simulink model "closed_loop_system_modal_kp_kv_robustness"  (R2022a)
settings: Solver=ode45  StartTime=0.0  StopTime=10.0  RelTol=1e-3  EnableMultiTasking=on
values from neighbouring files (symbols this model uses):
  Jpl = 0.0124    [lead_compensator.m]    (also in open_loop_complete_system_analysis.m; poles_placement_kp_kv.m; poles_placement_kp_kv_int.m)
  k = 1    [lead_compensator.m]    (also in poles_placement_kp_kv.m = place(openloop_modal_ss.a,openloop_modal_ss.b,lambda); poles_placement_kp_kv_int.m = place(openloop_modal_int_ss.a,openloop_modal_int_ss.b,lambda)
  km = 0.0235    [lead_compensator.m]    (also in open_loop_complete_system_analysis.m; poles_placement_kp_kv.m; poles_placement_kp_kv_int.m)
settings Model: Creator=c.ponzoni  LastModifiedBy=fades
settings SolverCC: AlgebraicLoopSolver=TrustRegion
settings DataIOCC: LimitDataPoints=on  SaveFormat=Array  ReturnWorkspaceOutputs=off
settings OptimizationCC: ExpressionDepthLimit=2147483647  LifeSpan=inf
settings DebuggingCC: UnderspecifiedInitializationDetection=Classic  MergeDetectMultiDrivingBlocksExec=none  UnconnectedInputMsg=warning  UnconnectedOutputMsg=warning  UnconnectedLineMsg=warning  StateNameClashWarn=warning  SFUnexpectedBacktrackingDiag=warning  SFNoUnconditionalDefaultTransitionDiag=warning  SFExecutionAtInitializationDiag=none  SFMachineParentedDataDiag=warning  ArithmeticOperatorsInVariantConditions=warning
settings HardwareCC: ProdBitPerPointer=32  ProdBitPerSizeT=32  ProdBitPerPtrDiffT=32  ProdLargestAtomicFloat=None  ProdIntDivRoundTo=Undefined  ProdEndianess=Unspecified  ProdWordSize=32  ProdHWDeviceType=32-bit Generic
settings ModelReferenceCC: PropagateSignalLabelsOutOfModel=off
settings SFSimCC: SimUseLocalCustomCode=off  CustomCodeUndefinedFunction=UseInterfaceOnly
settings RTWCC: RTWUseLocalCustomCode=off
settings CodeAppCC: StateflowObjectComments=on
settings GRTTargetCC: TargetLangStandard=C89/C90 (ANSI)
settings ConfigComp: CovMetricSettings=dw  CovSaveCumulativeToWorkspaceVar=on  CovSaveSingleToWorkspaceVar=on  CovExternalEMLEnable=off

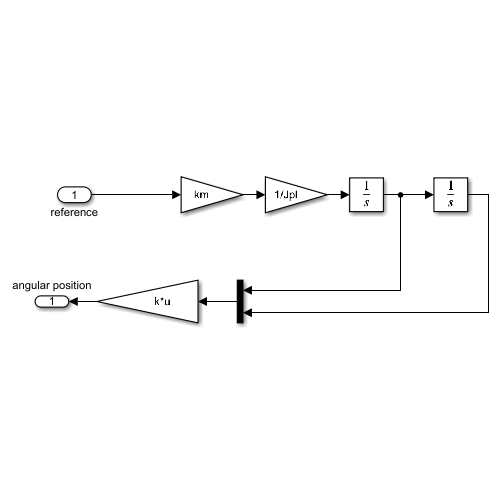
[thumbnail: Simulink's stored preview of the top-level diagram]
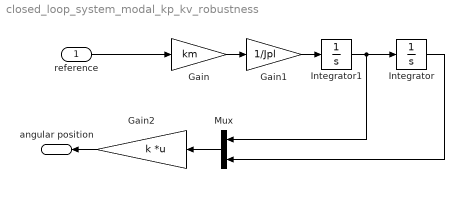
== system closed_loop_system_modal_kp_kv_robustness ==
  reference : Inport
  Gain : Gain  Gain=km  SaturateOnIntegerOverflow=on  OutDataTypeStr=Inherit: Same as input  ParamDataTypeStr=Inherit: Same as input
  Gain1 : Gain  Gain=1/Jpl  SaturateOnIntegerOverflow=on  OutDataTypeStr=Inherit: Same as input  ParamDataTypeStr=Inherit: Same as input
  Gain2 : Gain  Gain=k  Multiplication=Matrix(K*u)  SaturateOnIntegerOverflow=on  OutDataTypeStr=Inherit: Same as input  ParamDataTypeStr=Inherit: Same as input
  Integrator : Integrator
  Integrator1 : Integrator
  Mux : Mux  Inputs=2
  angular position : Outport  VectorParamsAs1DForOutWhenUnconnected=off
  wires:
  Integrator1/1 -> Mux/1, Integrator/1
  Gain1/1 -> Integrator1/1
  Gain/1 -> Gain1/1
  Integrator/1 -> Mux/2
  Mux/1 -> Gain2/1
  Gain2/1 -> angular position/1
  reference/1 -> Gain/1
